simulink model "Custom_PID"  (R2023b)
settings: Solver=VariableStepAuto  StartTime=0.0  StopTime=10.0  RelTol=1e-3

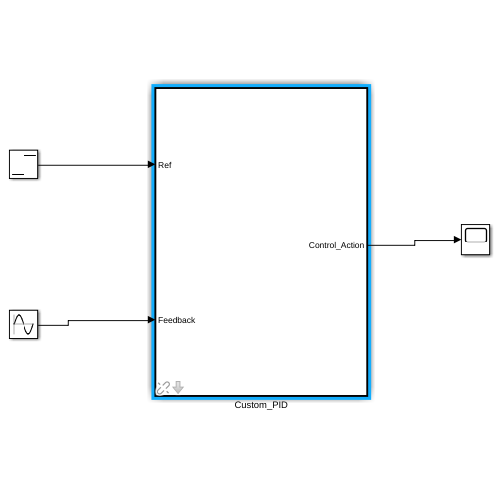
[thumbnail: Simulink's stored preview of the top-level diagram]
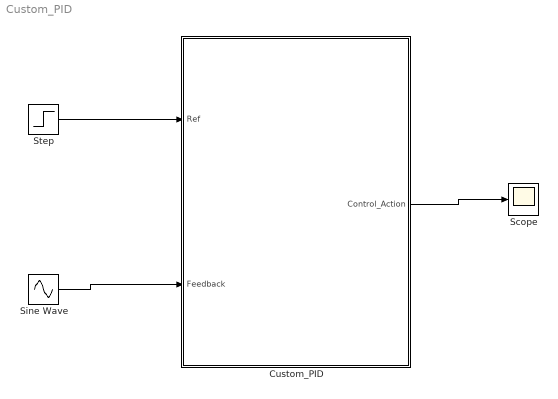
== system Custom_PID ==
  Custom_PID : Subsystem  AncestorBlock=Custom_PID/Custom_PID  TreatAsAtomicUnit=on  mask{Kp=1, Ki=0.1, Kd=2, IC=0}
      mask prompts: Kp "Proportional"; Ki "Integral"; Kd "Differential"; IC "Initial Condition"
      mask help:
      | Custom PID Control
      |
      | Propotional is the control Kp
      | Integral is the control Ki
      | Differential is the control Kd
  Scope : Scope
  Sine Wave : Sin  SampleTime=0
  Step : Step  SampleTime=0
  wires:
  Sine Wave/1 -> Custom_PID/2(Feedback)
  Step/1 -> Custom_PID/1(Ref)
  Custom_PID/1(Control_Action) -> Scope/1

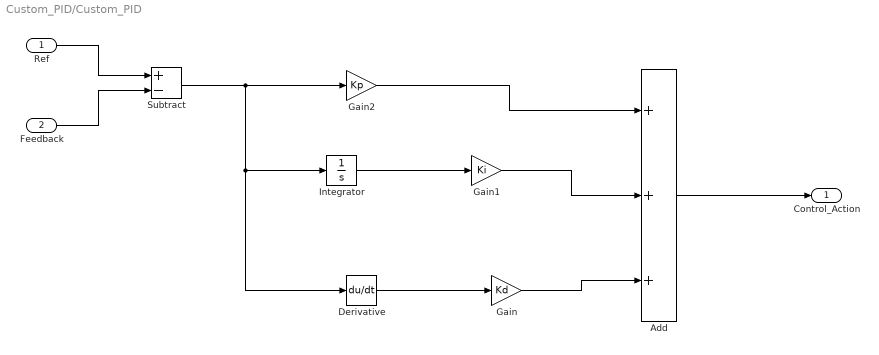
== system Custom_PID/Custom_PID ==
  Ref : Inport
  Feedback : Inport  Port=2
  Add : Sum  Inputs=+++
  Derivative : Derivative
  Gain : Gain  Gain=Kd
  Gain1 : Gain  Gain=Ki
  Gain2 : Gain  Gain=Kp
  Integrator : Integrator  InitialCondition=IC
  Subtract : Sum  Inputs=+-
  Control_Action : Outport
  wires:
  Ref/1 -> Subtract/1
  Add/1 -> Control_Action/1
  Subtract/1 -> Gain2/1, Derivative/1, Integrator/1
  Derivative/1 -> Gain/1
  Feedback/1 -> Subtract/2
  Gain2/1 -> Add/1
  Gain/1 -> Add/3
  Integrator/1 -> Gain1/1
  Gain1/1 -> Add/2
